simulink model "pratica_4"  (R2021b)
settings: Solver=VariableStepAuto  StartTime=0.0  StopTime=10.0  RelTol=1e-3
settings Model: Creator=julio-ribeiro  LastModifiedBy=julio-ribeiro

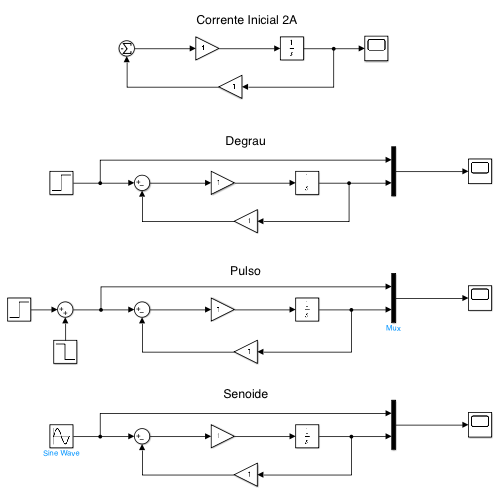
[thumbnail: Simulink's stored preview of the top-level diagram]
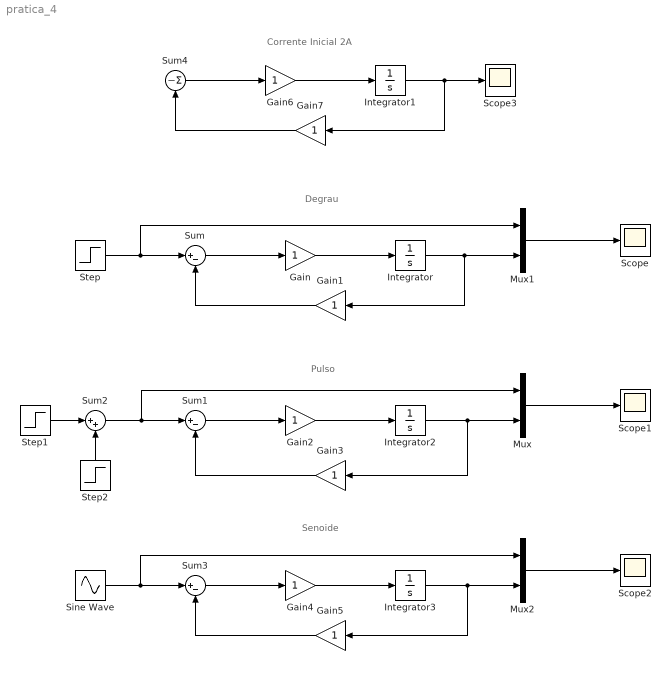
== system pratica_4 ==
  note: Senoide
  note: Pulso
  note: Degrau
  note: Corrente Inicial 2A
  Gain{,1..7} (8 alike) : Gain
  Integrator : Integrator
  Integrator1 : Integrator  InitialCondition=2
  Integrator2 : Integrator
  Integrator3 : Integrator
  Mux : Mux  Inputs=2
  Mux1 : Mux  Inputs=2
  Mux2 : Mux  Inputs=2
  Scope{,1..3} (4 alike) : Scope
  Sine Wave : Sin  Frequency=2  SampleTime=0
  Step : Step  SampleTime=0
  Step1 : Step  SampleTime=0
  Step2 : Step  Time=2  After=-1  SampleTime=0
  Sum : Sum  Inputs=|+-
  Sum1 : Sum  Inputs=|+-
  Sum2 : Sum  Inputs=|++
  Sum3 : Sum  Inputs=|+-
  Sum4 : Sum  Inputs=|-
  wires:
  Sum/1 -> Gain/1
  Gain1/1 -> Sum/2
  Step/1 -> Mux1/1, Sum/1
  Sum1/1 -> Gain2/1
  Gain3/1 -> Sum1/2
  Sum2/1 -> Mux/1, Sum1/1
  Step1/1 -> Sum2/1
  Step2/1 -> Sum2/2
  Mux/1 -> Scope1/1
  Mux1/1 -> Scope/1
  Sum3/1 -> Gain4/1
  Sine Wave/1 -> Mux2/1, Sum3/1
  Gain5/1 -> Sum3/2
  Mux2/1 -> Scope2/1
  Gain/1 -> Integrator/1
  Integrator/1 -> Gain1/1, Mux1/2
  Sum4/1 -> Gain6/1
  Integrator1/1 -> Scope3/1, Gain7/1
  Gain6/1 -> Integrator1/1
  Gain7/1 -> Sum4/1
  Integrator2/1 -> Gain3/1, Mux/2
  Gain2/1 -> Integrator2/1
  Gain4/1 -> Integrator3/1
  Integrator3/1 -> Gain5/1, Mux2/2
